simulink model "controller_subsystem"  (R2020b)
settings: Solver=VariableStepAuto  StartTime=0.0  StopTime=10.0  RelTol=1e-3
undefined symbols (not defined in the file): pitchRateKd, pitchRateKi, pitchRateKp, rollRateKd, rollRateKi, rollRateKp, u1, u2, u3, u4, xKd, xKi, xKp, yawRateKd, yawRateKi, yawRateKp, yKd, yKi, yKp, zKd, zKi, zKp
settings Model: Creator=jbmic  LastModifiedBy=jbmic

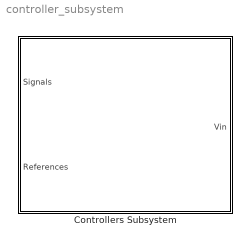
== system controller_subsystem ==
  Controllers Subsystem : Subsystem

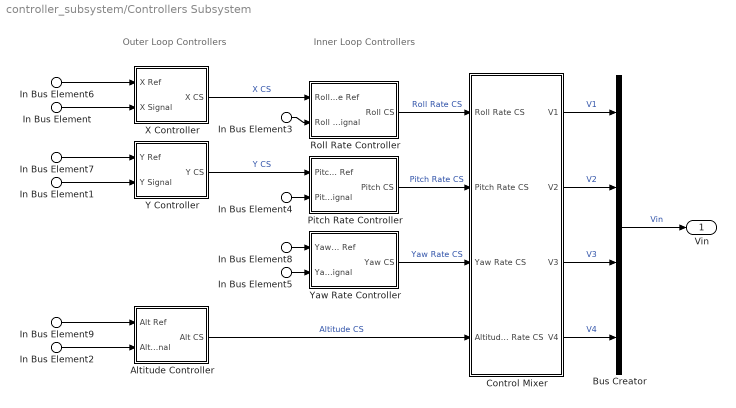
== system controller_subsystem/Controllers Subsystem ==
  note: Inner Loop Controllers
  note: Outer Loop Controllers
  In Bus Element : Inport  PortName=Signals  Element=X
  In Bus Element1 : Inport  PortName=Signals  Element=Y
  In Bus Element2 : Inport  PortName=Signals  Element=Z
  In Bus Element3 : Inport  PortName=Signals  Element=Roll
  In Bus Element4 : Inport  PortName=Signals  Element=Pitch
  In Bus Element5 : Inport  PortName=Signals  Element=Yaw
  In Bus Element6 : Inport  Port=2  PortName=References  Element=X Ref
  In Bus Element7 : Inport  Port=2  PortName=References  Element=Y Ref
  In Bus Element8 : Inport  Port=2  PortName=References  Element=Yaw Rate Ref
  In Bus Element9 : Inport  Port=2  PortName=References  Element=Z Ref
  Altitude Controller : Subsystem
  Bus Creator : BusCreator  Inputs=4
  Control Mixer : Subsystem
  Pitch Rate Controller : Subsystem
  Roll Rate Controller : Subsystem
  X Controller : Subsystem
  Y Controller : Subsystem
  Yaw Rate Controller : Subsystem
  Vin : Outport
  wires:
  In Bus Element9/1 -> Altitude Controller/1(Alt Ref)
  In Bus Element6/1 -> X Controller/1(X Ref)
  Control Mixer/3(V3) -> Bus Creator/3  "V3"
  In Bus Element8/1 -> Yaw Rate Controller/1(Yaw Rate Ref)
  Yaw Rate Controller/1(Yaw CS) -> Control Mixer/3(Yaw Rate CS)  "Yaw Rate CS"
  In Bus Element7/1 -> Y Controller/1(Y Ref)
  Altitude Controller/1(Alt CS) -> Control Mixer/4(Altitude Rate CS)  "Altitude CS"
  X Controller/1(X CS) -> Roll Rate Controller/1(Roll Rate Ref)  "X CS"
  Y Controller/1(Y CS) -> Pitch Rate Controller/1(Pitch Rate Ref)  "Y CS"
  Pitch Rate Controller/1(Pitch CS) -> Control Mixer/2(Pitch Rate CS)  "Pitch Rate CS"
  Control Mixer/2(V2) -> Bus Creator/2  "V2"
  Roll Rate Controller/1(Roll CS) -> Control Mixer/1(Roll Rate CS)  "Roll Rate CS"
  Bus Creator/1 -> Vin/1  "Vin"
  Control Mixer/4(V4) -> Bus Creator/4  "V4"
  Control Mixer/1(V1) -> Bus Creator/1  "V1"
  In Bus Element/1 -> X Controller/2(X Signal)
  In Bus Element1/1 -> Y Controller/2(Y Signal)
  In Bus Element2/1 -> Altitude Controller/2(Alt Signal)
  In Bus Element3/1 -> Roll Rate Controller/2(Roll Rate Signal)
  In Bus Element4/1 -> Pitch Rate Controller/2(Pitch Rate Signal)
  In Bus Element5/1 -> Yaw Rate Controller/2(Yaw Rate Signal)

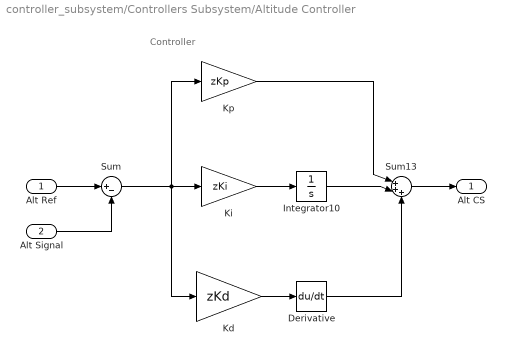
== system controller_subsystem/Controllers Subsystem/Altitude Controller ==
  note: Controller
  Alt Ref : Inport
  Alt Signal : Inport  Port=2
  Derivative : Derivative
  Integrator10 : Integrator
  "Kd " : Gain  Gain=zKd
  Ki : Gain  Gain=zKi
  Kp : Gain  Gain=zKp
  Sum : Sum  Inputs=|+-
  Sum13 : Sum  Inputs=|+++
  Alt CS : Outport
  wires:
  Derivative/1 -> Sum13/3
  Ki/1 -> Integrator10/1
  Integrator10/1 -> Sum13/2
  Kp/1 -> Sum13/1
  "Kd "/1 -> Derivative/1
  Sum13/1 -> Alt CS/1
  Alt Ref/1 -> Sum/1
  Alt Signal/1 -> Sum/2
  Sum/1 -> Kp/1, "Kd "/1, Ki/1

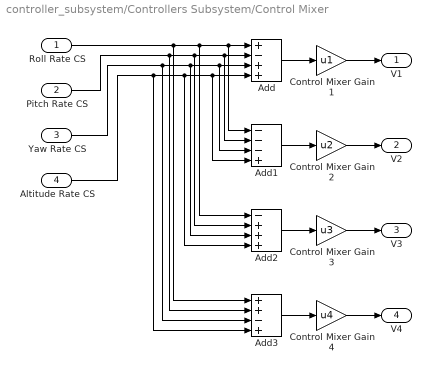
== system controller_subsystem/Controllers Subsystem/Control Mixer ==
  Roll Rate CS : Inport
  Pitch Rate CS : Inport  Port=2
  Yaw Rate CS : Inport  Port=3
  Altitude Rate CS : Inport  Port=4
  Add : Sum  Inputs=+-++
  Add1 : Sum  Inputs=---+
  Add2 : Sum  Inputs=-+++
  Add3 : Sum  Inputs=++-+
  Control Mixer Gain 1 : Gain  Gain=u1
  Control Mixer Gain 2 : Gain  Gain=u2
  Control Mixer Gain 3 : Gain  Gain=u3
  Control Mixer Gain 4 : Gain  Gain=u4
  V1 : Outport
  V2 : Outport  Port=2
  V3 : Outport  Port=3
  V4 : Outport  Port=4
  wires:
  Add/1 -> Control Mixer Gain 1/1
  Add1/1 -> Control Mixer Gain 2/1
  Add3/1 -> Control Mixer Gain 4/1
  Add2/1 -> Control Mixer Gain 3/1
  Control Mixer Gain 1/1 -> V1/1
  Control Mixer Gain 2/1 -> V2/1
  Control Mixer Gain 3/1 -> V3/1
  Control Mixer Gain 4/1 -> V4/1
  Roll Rate CS/1 -> Add1/1, Add/1, Add2/1, Add3/1
  Pitch Rate CS/1 -> Add1/2, Add/2, Add2/2, Add3/2
  Yaw Rate CS/1 -> Add3/3, Add1/3, Add/3, Add2/3
  Altitude Rate CS/1 -> Add2/4, Add1/4, Add/4, Add3/4

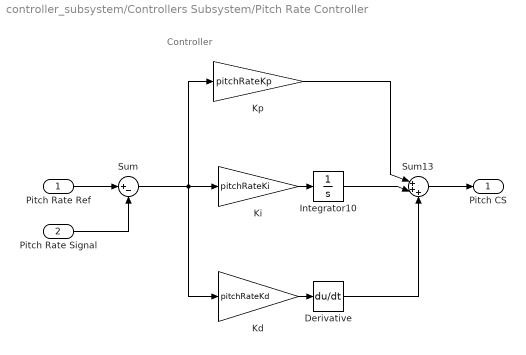
== system controller_subsystem/Controllers Subsystem/Pitch Rate Controller ==
  note: Controller
  Pitch Rate Ref : Inport
  Pitch Rate Signal : Inport  Port=2
  Derivative : Derivative
  Integrator10 : Integrator
  Kd : Gain  Gain=pitchRateKd
  Ki : Gain  Gain=pitchRateKi
  Kp : Gain  Gain=pitchRateKp
  Sum : Sum  Inputs=|+-
  Sum13 : Sum  Inputs=|+++
  Pitch CS : Outport
  wires:
  Derivative/1 -> Sum13/3
  Ki/1 -> Integrator10/1
  Integrator10/1 -> Sum13/2
  Kp/1 -> Sum13/1
  Kd/1 -> Derivative/1
  Sum13/1 -> Pitch CS/1
  Pitch Rate Ref/1 -> Sum/1
  Pitch Rate Signal/1 -> Sum/2
  Sum/1 -> Kd/1, Ki/1, Kp/1

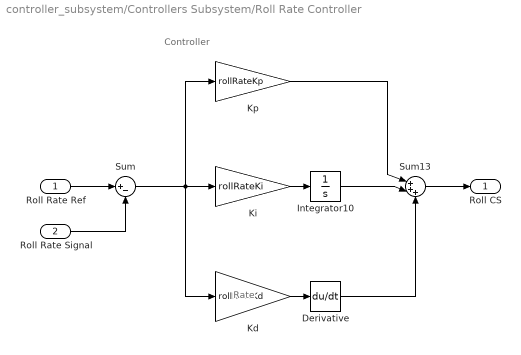
== system controller_subsystem/Controllers Subsystem/Roll Rate Controller ==
  note: Rate
  note: Controller
  Roll Rate Ref : Inport
  Roll Rate Signal : Inport  Port=2
  Derivative : Derivative
  Integrator10 : Integrator
  Kd : Gain  Gain=rollRateKd
  Ki : Gain  Gain=rollRateKi
  Kp : Gain  Gain=rollRateKp
  Sum : Sum  Inputs=|+-
  Sum13 : Sum  Inputs=|+++
  Roll CS : Outport
  wires:
  Derivative/1 -> Sum13/3
  Ki/1 -> Integrator10/1
  Integrator10/1 -> Sum13/2
  Kp/1 -> Sum13/1
  Kd/1 -> Derivative/1
  Sum13/1 -> Roll CS/1
  Roll Rate Ref/1 -> Sum/1
  Roll Rate Signal/1 -> Sum/2
  Sum/1 -> Ki/1, Kp/1, Kd/1

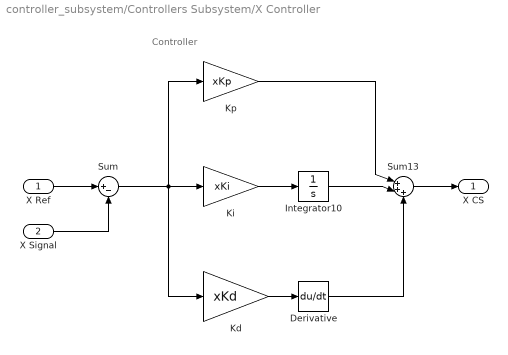
== system controller_subsystem/Controllers Subsystem/X Controller ==
  note: Controller
  X Ref : Inport
  X Signal : Inport  Port=2
  Derivative : Derivative
  Integrator10 : Integrator
  Kd : Gain  Gain=xKd
  Ki : Gain  Gain=xKi
  Kp : Gain  Gain=xKp
  Sum : Sum  Inputs=|+-
  Sum13 : Sum  Inputs=|+++
  X CS : Outport
  wires:
  Derivative/1 -> Sum13/3
  Ki/1 -> Integrator10/1
  Integrator10/1 -> Sum13/2
  Kp/1 -> Sum13/1
  Kd/1 -> Derivative/1
  Sum13/1 -> X CS/1
  X Ref/1 -> Sum/1
  X Signal/1 -> Sum/2
  Sum/1 -> Kd/1, Kp/1, Ki/1

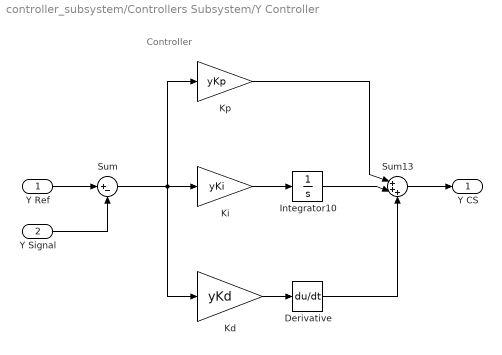
== system controller_subsystem/Controllers Subsystem/Y Controller ==
  note: Controller
  Y Ref : Inport
  Y Signal : Inport  Port=2
  Derivative : Derivative
  Integrator10 : Integrator
  Kd : Gain  Gain=yKd
  Ki : Gain  Gain=yKi
  Kp : Gain  Gain=yKp
  Sum : Sum  Inputs=|+-
  Sum13 : Sum  Inputs=|+++
  Y CS : Outport
  wires:
  Derivative/1 -> Sum13/3
  Ki/1 -> Integrator10/1
  Integrator10/1 -> Sum13/2
  Kp/1 -> Sum13/1
  Kd/1 -> Derivative/1
  Sum13/1 -> Y CS/1
  Y Ref/1 -> Sum/1
  Y Signal/1 -> Sum/2
  Sum/1 -> Kd/1, Kp/1, Ki/1

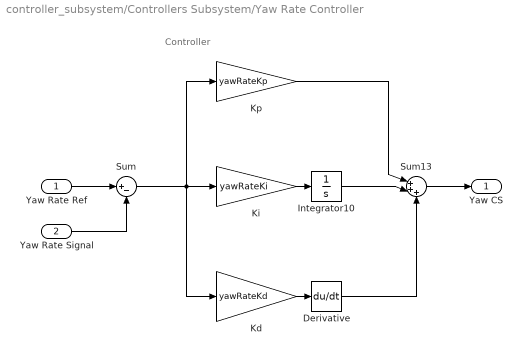
== system controller_subsystem/Controllers Subsystem/Yaw Rate Controller ==
  note: Controller
  Yaw Rate Ref : Inport
  Yaw Rate Signal : Inport  Port=2
  Derivative : Derivative
  Integrator10 : Integrator
  Kd : Gain  Gain=yawRateKd
  Ki : Gain  Gain=yawRateKi
  Kp : Gain  Gain=yawRateKp
  Sum : Sum  Inputs=|+-
  Sum13 : Sum  Inputs=|+++
  Yaw CS : Outport
  wires:
  Derivative/1 -> Sum13/3
  Ki/1 -> Integrator10/1
  Integrator10/1 -> Sum13/2
  Kp/1 -> Sum13/1
  Kd/1 -> Derivative/1
  Sum13/1 -> Yaw CS/1
  Yaw Rate Ref/1 -> Sum/1
  Yaw Rate Signal/1 -> Sum/2
  Sum/1 -> Ki/1, Kp/1, Kd/1
